simulink model "ALL_JP360_DBW_V6_5_1103"  (R2022a)
settings: Solver=FixedStepAuto  StartTime=0.0  StopTime=inf  FixedStep=0.01  RelTol=1e-3  EnableMultiTasking=on
model workspace (MAT data in the model file):
  g = 9.8
undefined symbols (not defined in the file or in its folder): canChannel, delta_v_p, IPM_Line_C0, IPM_Line_C1, IPM_Line_C2, IPM_Line_C3, M, M_p, MRR_ObjDistX, MRR_ObjDistY, MRR_ObjFusionCamID, MRR_ObjFusionSig, MRR_ObjID, MRR_ObjRelVelX, MRR_ObjRelVelY, MRR_ObjType, MRR_ObjUpdFlg, none, obj_vaild, untracktime, V, videoinput
libraries: canfdmsglib x230, canfdlib x76, slpidlib x24, simulink x18, dspstat3 x14, ctrlSharedLib x1, simulink_extras x1, imaqlib x1, realtime_pacer_lib x1, dspvision x1, visionsinks x1
(part 25 of 55)

== system ALL_JP360_DBW_V6_5_1103/MsgFromCAN/SRR_ADCU_MsgFromCAN/SRR_ADCU_FRR_OBJPos1_0x1A3 ==
  SRR_ADCU_FRR_OBJPos1_0x1A3FromInData : Inport  OutDataTypeStr=Bus:CAN_FD_MESSAGE_BUS
  Bus Creator : BusCreator  Inputs=42  OutDataTypeStr=Bus:SRR_ADCU_FRR_OBJPos1_0x1A3  NonVirtualBus=on
  CAN FD Unpack : canfdmsglib/CAN FD Unpack  CANdbFile=V363 SRR Private CAN-V1.3.dbc  MsgList=(none)  MsgName=FRR_OBJPos1_0x1A3  ProtocolMode=CAN FD  MsgIDType=Standard (11-bit identifier)  MsgIdentifier=419  MsgLength=48  SignalInfo={'FRR_CRCCheck_0x1A3','376','16','BE','unsigned','Standard','0','1','0','0','65535';'FRR_OBJ1_Dx','79','13','BE','unsigned','Standard','0','0.0625','-256','-256','255.938';'FRR_OBJ1_Dy','60','11','BE','unsigned','Standard','0','0.125','-128','-128','127.875';'FRR_OBJ1_ExistProb','112','6','BE','unsigned','Standard','0','2','0','0','100';'FRR_OBJ1_HeadingAngle','55','10','BE','unsigned','Standard','0','0.01','-3.14','-3.14','3.14';'FRR_OBJ1_Height','26','9','BE','unsigned','Standard','0','0.01','0','0','5.11';'FRR_OBJ1_Length','33','9','BE','unsigned','Standard','0','0.05','0','0','25.5';'FRR_OBJ1_Measured','126','2','BE','unsigned','Standard','0','1','0','0','3';'FRR_OBJ1_Motion_Status','162','3','BE','unsigned','Standard','0','1','0','0','7';'FRR_OBJ1_ObstacleProb','120','6','BE','unsigned','Standard','0','2','0','0','100';'FRR_OBJ1_RefPointDx','144','13','BE','unsigned','Standard','0','0.0625','-256','-256','255.938';'FRR_OBJ1_RefPointDy','141','11','BE','unsigned','Standard','0','0.125','-128','-128','127.875';'FRR_OBJ1_RefPointLoc','157','3','BE','unsigned','Standard','0','1','0','0','7';'FRR_OBJ1_RelAx','118','9','BE','unsigned','Standard','0','0.0625','-16','-16','15.9375';'FRR_OBJ1_RelAy','111','10','BE','unsigned','Standard','0','0.03125','-16','-16','15.9688';'FRR_OBJ1_RelVx','89','12','BE','unsigned','Standard','0','0.0625','-128','-128','127.938';'FRR_OBJ1_RelVy','85','10','BE','unsigned','Standard','0','0.125','-64','-64','63.875';'FRR_OBJ1_Track_Age','165','8','BE','unsigned','Standard','0','1','0','0','255';'FRR_OBJ1_Track_ID','1','7','BE','unsigned','Standard','0','1','0','0','127';'FRR_OBJ1_Type','14','3','BE','unsigned','Standard','0','1','0','0','7';'FRR_OBJ1_Width','19','11','BE','unsigned','Standard','0','0.01','0','0','12';'FRR_OBJ2_Dx','247','13','BE','unsigned','Standard','0','0.0625','-256','-256','255.938';'FRR_OBJ2_Dy','228','11','BE','unsigned','Standard','0','0.125','-128','-128','127.875';'FRR_OBJ2_ExistProb','280','6','BE','unsigned','Standard','0','2','0','0','100';'FRR_OBJ2_HeadingAngle','223','10','BE','unsigned','Standard','0','0.01','-3.14','-3.14','3.14';'FRR_OBJ2_Height','194','9','BE','unsigned','Standard','0','0.01','0','0','5.11';'FRR_OBJ2_Length','201','9','BE','unsigned','Standard','0','0.05','0','0','25.5';'FRR_OBJ2_Measured','294','2','BE','unsigned','Standard','0','1','0','0','3';'FRR_OBJ2_Motion_Status','330','3','BE','unsigned','Standard','0','1','0','0','7';'FRR_OBJ2_ObstacleProb','288','6','BE','unsigned','Standard','0','2','0','0','100';'FRR_OBJ2_RefPointDx','312','13','BE','unsigned','Standard','0','0.0625','-256','-256','255.938';'FRR_OBJ2_RefPointDy','309','11','BE','unsigned','Standard','0','0.125','-128','-128','127.875';'FRR_OBJ2_RefPointLoc','325','3','BE','unsigned','Standard','0','1','0','0','7';'FRR_OBJ2_RelAx','286','9','BE','unsigned','Standard','0','0.0625','-16','-16','15.9375';'FRR_OBJ2_RelAy','279','10','BE','unsigned','Standard','0','0.03125','-16','-16','15.9688';'FRR_OBJ2_RelVx','257','12','BE','unsigned','Standard','0','0.0625','-128','-128','127.938';'FRR_OBJ2_RelVy','253','10','BE','unsigned','Standard','0','0.125','-64','-64','63.875';'FRR_OBJ2_Track_Age','333','8','BE','unsigned','Standard','0','1','0','0','255';'FRR_OBJ2_Track_ID','169','7','BE','unsigned','Standard','0','1','0','0','127';'FRR_OBJ2_Type','182','3','BE','unsigned','Standard','0','1','0','0','7';'FRR_OBJ2_Width','187','11','BE','unsigned','Standard','0','0.01','0','0','12';'FRR_RollingCounter_0x1A3','360','4','BE','unsigned','Standard','0','1','0','0','15'}  IDPort=off  TimestampPort=off  ErrorPort=off  RemotePort=off  LengthPort=off  StatusPort=off  BRSPort=off  ESIPort=off  DLCPort=off  ApplyMinMax=off
      settings: SourceProductBaseCode=ME,XP,VN  DataFormat=CANdb specified signals
  Data Type Conversion1 : DataTypeConversion  OutDataTypeStr=uint16  SaturateOnIntegerOverflow=off  RndMeth=Floor
  Data Type Conversion{4,8..10,13,19..20,24,28..30,33,39..40,42} (15 alike) : DataTypeConversion  OutDataTypeStr=int8  SaturateOnIntegerOverflow=off  RndMeth=Floor
  Data Type Conversion{2..3,5..7,11..12,14..17,21..23,25..27,31..32,34..37,41} (24 alike) : DataTypeConversion  OutDataTypeStr=single  SaturateOnIntegerOverflow=off  RndMeth=Floor
  Data Type Conversion18 : DataTypeConversion  OutDataTypeStr=uint8  SaturateOnIntegerOverflow=off  RndMeth=Floor
  Data Type Conversion38 : DataTypeConversion  OutDataTypeStr=uint8  SaturateOnIntegerOverflow=off  RndMeth=Floor
  SRR_ADCU_FRR_OBJPos1_0x1A3FromOutData : Outport  OutDataTypeStr=Bus:SRR_ADCU_FRR_OBJPos1_0x1A3
  wires:
  CAN FD Unpack/1 -> Data Type Conversion1/1
  CAN FD Unpack/2 -> Data Type Conversion2/1
  CAN FD Unpack/3 -> Data Type Conversion3/1
  CAN FD Unpack/4 -> Data Type Conversion4/1
  CAN FD Unpack/5 -> Data Type Conversion5/1
  CAN FD Unpack/6 -> Data Type Conversion6/1
  CAN FD Unpack/7 -> Data Type Conversion7/1
  CAN FD Unpack/8 -> Data Type Conversion8/1
  CAN FD Unpack/9 -> Data Type Conversion9/1
  CAN FD Unpack/10 -> Data Type Conversion10/1
  CAN FD Unpack/11 -> Data Type Conversion11/1
  CAN FD Unpack/12 -> Data Type Conversion12/1
  CAN FD Unpack/13 -> Data Type Conversion13/1
  CAN FD Unpack/14 -> Data Type Conversion14/1
  CAN FD Unpack/15 -> Data Type Conversion15/1
  CAN FD Unpack/16 -> Data Type Conversion16/1
  CAN FD Unpack/17 -> Data Type Conversion17/1
  CAN FD Unpack/18 -> Data Type Conversion18/1
  CAN FD Unpack/19 -> Data Type Conversion19/1
  CAN FD Unpack/20 -> Data Type Conversion20/1
  CAN FD Unpack/21 -> Data Type Conversion21/1
  CAN FD Unpack/22 -> Data Type Conversion22/1
  CAN FD Unpack/23 -> Data Type Conversion23/1
  CAN FD Unpack/24 -> Data Type Conversion24/1
  CAN FD Unpack/25 -> Data Type Conversion25/1
  CAN FD Unpack/26 -> Data Type Conversion26/1
  CAN FD Unpack/27 -> Data Type Conversion27/1
  CAN FD Unpack/28 -> Data Type Conversion28/1
  CAN FD Unpack/29 -> Data Type Conversion29/1
  CAN FD Unpack/30 -> Data Type Conversion30/1
  CAN FD Unpack/31 -> Data Type Conversion31/1
  CAN FD Unpack/32 -> Data Type Conversion32/1
  CAN FD Unpack/33 -> Data Type Conversion33/1
  CAN FD Unpack/34 -> Data Type Conversion34/1
  CAN FD Unpack/35 -> Data Type Conversion35/1
  CAN FD Unpack/36 -> Data Type Conversion36/1
  CAN FD Unpack/37 -> Data Type Conversion37/1
  CAN FD Unpack/38 -> Data Type Conversion38/1
  CAN FD Unpack/39 -> Data Type Conversion39/1
  CAN FD Unpack/40 -> Data Type Conversion40/1
  CAN FD Unpack/41 -> Data Type Conversion41/1
  CAN FD Unpack/42 -> Data Type Conversion42/1
  Data Type Conversion1/1 -> Bus Creator/1  "FRR_CRCCheck_0x1A3"
  Data Type Conversion2/1 -> Bus Creator/2  "FRR_OBJ1_Dx"
  Data Type Conversion3/1 -> Bus Creator/3  "FRR_OBJ1_Dy"
  Data Type Conversion4/1 -> Bus Creator/4  "FRR_OBJ1_ExistProb"
  Data Type Conversion5/1 -> Bus Creator/5  "FRR_OBJ1_HeadingAngle"
  Data Type Conversion6/1 -> Bus Creator/6  "FRR_OBJ1_Height"
  Data Type Conversion7/1 -> Bus Creator/7  "FRR_OBJ1_Length"
  Data Type Conversion8/1 -> Bus Creator/8  "FRR_OBJ1_Measured"
  Data Type Conversion9/1 -> Bus Creator/9  "FRR_OBJ1_Motion_Status"
  Data Type Conversion10/1 -> Bus Creator/10  "FRR_OBJ1_ObstacleProb"
  Data Type Conversion11/1 -> Bus Creator/11  "FRR_OBJ1_RefPointDx"
  Data Type Conversion12/1 -> Bus Creator/12  "FRR_OBJ1_RefPointDy"
  Data Type Conversion13/1 -> Bus Creator/13  "FRR_OBJ1_RefPointLoc"
  Data Type Conversion14/1 -> Bus Creator/14  "FRR_OBJ1_RelAx"
  Data Type Conversion15/1 -> Bus Creator/15  "FRR_OBJ1_RelAy"
  Data Type Conversion16/1 -> Bus Creator/16  "FRR_OBJ1_RelVx"
  Data Type Conversion17/1 -> Bus Creator/17  "FRR_OBJ1_RelVy"
  Data Type Conversion18/1 -> Bus Creator/18  "FRR_OBJ1_Track_Age"
  Data Type Conversion19/1 -> Bus Creator/19  "FRR_OBJ1_Track_ID"
  Data Type Conversion20/1 -> Bus Creator/20  "FRR_OBJ1_Type"
  Data Type Conversion21/1 -> Bus Creator/21  "FRR_OBJ1_Width"
  Data Type Conversion22/1 -> Bus Creator/22  "FRR_OBJ2_Dx"
  Data Type Conversion23/1 -> Bus Creator/23  "FRR_OBJ2_Dy"
  Data Type Conversion24/1 -> Bus Creator/24  "FRR_OBJ2_ExistProb"
  Data Type Conversion25/1 -> Bus Creator/25  "FRR_OBJ2_HeadingAngle"
  Data Type Conversion26/1 -> Bus Creator/26  "FRR_OBJ2_Height"
  Data Type Conversion27/1 -> Bus Creator/27  "FRR_OBJ2_Length"
  Data Type Conversion28/1 -> Bus Creator/28  "FRR_OBJ2_Measured"
  Data Type Conversion29/1 -> Bus Creator/29  "FRR_OBJ2_Motion_Status"
  Data Type Conversion30/1 -> Bus Creator/30  "FRR_OBJ2_ObstacleProb"
  Data Type Conversion31/1 -> Bus Creator/31  "FRR_OBJ2_RefPointDx"
  Data Type Conversion32/1 -> Bus Creator/32  "FRR_OBJ2_RefPointDy"
  Data Type Conversion33/1 -> Bus Creator/33  "FRR_OBJ2_RefPointLoc"
  Data Type Conversion34/1 -> Bus Creator/34  "FRR_OBJ2_RelAx"
  Data Type Conversion35/1 -> Bus Creator/35  "FRR_OBJ2_RelAy"
  Data Type Conversion36/1 -> Bus Creator/36  "FRR_OBJ2_RelVx"
  Data Type Conversion37/1 -> Bus Creator/37  "FRR_OBJ2_RelVy"
  Data Type Conversion38/1 -> Bus Creator/38  "FRR_OBJ2_Track_Age"
  Data Type Conversion39/1 -> Bus Creator/39  "FRR_OBJ2_Track_ID"
  Data Type Conversion40/1 -> Bus Creator/40  "FRR_OBJ2_Type"
  Data Type Conversion41/1 -> Bus Creator/41  "FRR_OBJ2_Width"
  Data Type Conversion42/1 -> Bus Creator/42  "FRR_RollingCounter_0x1A3"
  Bus Creator/1 -> SRR_ADCU_FRR_OBJPos1_0x1A3FromOutData/1  "SRR_ADCU_FRR_OBJPos1_0x1A3FromOutData"
  SRR_ADCU_FRR_OBJPos1_0x1A3FromInData/1 -> CAN FD Unpack/1  "SRR_ADCU_FRR_OBJPos1_0x1A3FromInData"

== system ALL_JP360_DBW_V6_5_1103/MsgFromCAN/SRR_ADCU_MsgFromCAN/SRR_ADCU_FRR_OBJPos2_0x1A4 ==
  SRR_ADCU_FRR_OBJPos2_0x1A4FromInData : Inport  OutDataTypeStr=Bus:CAN_FD_MESSAGE_BUS
  Bus Creator : BusCreator  Inputs=42  OutDataTypeStr=Bus:SRR_ADCU_FRR_OBJPos2_0x1A4  NonVirtualBus=on
  CAN FD Unpack : canfdmsglib/CAN FD Unpack  CANdbFile=V363 SRR Private CAN-V1.3.dbc  MsgList=(none)  MsgName=FRR_OBJPos2_0x1A4  ProtocolMode=CAN FD  MsgIDType=Standard (11-bit identifier)  MsgIdentifier=420  MsgLength=48  SignalInfo={'FRR_CRCCheck_0x1A4','376','16','BE','unsigned','Standard','0','1','0','0','65535';'FRR_OBJ3_Dx','79','13','BE','unsigned','Standard','0','0.0625','-256','-256','255.938';'FRR_OBJ3_Dy','60','11','BE','unsigned','Standard','0','0.125','-128','-128','127.875';'FRR_OBJ3_ExistProb','112','6','BE','unsigned','Standard','0','2','0','0','100';'FRR_OBJ3_HeadingAngle','55','10','BE','unsigned','Standard','0','0.01','-3.14','-3.14','3.14';'FRR_OBJ3_Height','26','9','BE','unsigned','Standard','0','0.01','0','0','5.11';'FRR_OBJ3_Length','33','9','BE','unsigned','Standard','0','0.05','0','0','25.5';'FRR_OBJ3_Measured','126','2','BE','unsigned','Standard','0','1','0','0','3';'FRR_OBJ3_Motion_Status','162','3','BE','unsigned','Standard','0','1','0','0','7';'FRR_OBJ3_ObstacleProb','120','6','BE','unsigned','Standard','0','2','0','0','100';'FRR_OBJ3_RefPointDx','144','13','BE','unsigned','Standard','0','0.0625','-256','-256','255.938';'FRR_OBJ3_RefPointDy','141','11','BE','unsigned','Standard','0','0.125','-128','-128','127.875';'FRR_OBJ3_RefPointLoc','157','3','BE','unsigned','Standard','0','1','0','0','7';'FRR_OBJ3_RelAx','118','9','BE','unsigned','Standard','0','0.0625','-16','-16','15.9375';'FRR_OBJ3_RelAy','111','10','BE','unsigned','Standard','0','0.03125','-16','-16','15.9688';'FRR_OBJ3_RelVx','89','12','BE','unsigned','Standard','0','0.0625','-128','-128','127.938';'FRR_OBJ3_RelVy','85','10','BE','unsigned','Standard','0','0.125','-64','-64','63.875';'FRR_OBJ3_Track_Age','165','8','BE','unsigned','Standard','0','1','0','0','255';'FRR_OBJ3_Track_ID','1','7','BE','unsigned','Standard','0','1','0','0','127';'FRR_OBJ3_Type','14','3','BE','unsigned','Standard','0','1','0','0','7';'FRR_OBJ3_Width','19','11','BE','unsigned','Standard','0','0.01','0','0','12';'FRR_OBJ4_Dx','247','13','BE','unsigned','Standard','0','0.0625','-256','-256','255.938';'FRR_OBJ4_Dy','228','11','BE','unsigned','Standard','0','0.125','-128','-128','127.875';'FRR_OBJ4_ExistProb','280','6','BE','unsigned','Standard','0','2','0','0','100';'FRR_OBJ4_HeadingAngle','223','10','BE','unsigned','Standard','0','0.01','-3.14','-3.14','3.14';'FRR_OBJ4_Height','194','9','BE','unsigned','Standard','0','0.01','0','0','5.11';'FRR_OBJ4_Length','201','9','BE','unsigned','Standard','0','0.05','0','0','25.5';'FRR_OBJ4_Measured','294','2','BE','unsigned','Standard','0','1','0','0','3';'FRR_OBJ4_Motion_Status','330','3','BE','unsigned','Standard','0','1','0','0','7';'FRR_OBJ4_ObstacleProb','288','6','BE','unsigned','Standard','0','2','0','0','100';'FRR_OBJ4_RefPointDx','312','13','BE','unsigned','Standard','0','0.0625','-256','-256','255.938';'FRR_OBJ4_RefPointDy','309','11','BE','unsigned','Standard','0','0.125','-128','-128','127.875';'FRR_OBJ4_RefPointLoc','325','3','BE','unsigned','Standard','0','1','0','0','7';'FRR_OBJ4_RelAx','286','9','BE','unsigned','Standard','0','0.0625','-16','-16','15.9375';'FRR_OBJ4_RelAy','279','10','BE','unsigned','Standard','0','0.03125','-16','-16','15.9688';'FRR_OBJ4_RelVx','257','12','BE','unsigned','Standard','0','0.0625','-128','-128','127.938';'FRR_OBJ4_RelVy','253','10','BE','unsigned','Standard','0','0.125','-64','-64','63.875';'FRR_OBJ4_Track_Age','333','8','BE','unsigned','Standard','0','1','0','0','255';'FRR_OBJ4_Track_ID','169','7','BE','unsigned','Standard','0','1','0','0','127';'FRR_OBJ4_Type','182','3','BE','unsigned','Standard','0','1','0','0','7';'FRR_OBJ4_Width','187','11','BE','unsigned','Standard','0','0.01','0','0','12';'FRR_RollingCounter_0x1A4','360','4','BE','unsigned','Standard','0','1','0','0','15'}  IDPort=off  TimestampPort=off  ErrorPort=off  RemotePort=off  LengthPort=off  StatusPort=off  BRSPort=off  ESIPort=off  DLCPort=off  ApplyMinMax=off
      settings: SourceProductBaseCode=ME,XP,VN  DataFormat=CANdb specified signals
  Data Type Conversion1 : DataTypeConversion  OutDataTypeStr=uint16  SaturateOnIntegerOverflow=off  RndMeth=Floor
  Data Type Conversion{4,8..10,13,19..20,24,28..30,33,39..40,42} (15 alike) : DataTypeConversion  OutDataTypeStr=int8  SaturateOnIntegerOverflow=off  RndMeth=Floor
  Data Type Conversion{2..3,5..7,11..12,14..17,21..23,25..27,31..32,34..37,41} (24 alike) : DataTypeConversion  OutDataTypeStr=single  SaturateOnIntegerOverflow=off  RndMeth=Floor
  Data Type Conversion18 : DataTypeConversion  OutDataTypeStr=uint8  SaturateOnIntegerOverflow=off  RndMeth=Floor
  Data Type Conversion38 : DataTypeConversion  OutDataTypeStr=uint8  SaturateOnIntegerOverflow=off  RndMeth=Floor
  SRR_ADCU_FRR_OBJPos2_0x1A4FromOutData : Outport  OutDataTypeStr=Bus:SRR_ADCU_FRR_OBJPos2_0x1A4
  wires:
  CAN FD Unpack/1 -> Data Type Conversion1/1
  CAN FD Unpack/2 -> Data Type Conversion2/1
  CAN FD Unpack/3 -> Data Type Conversion3/1
  CAN FD Unpack/4 -> Data Type Conversion4/1
  CAN FD Unpack/5 -> Data Type Conversion5/1
  CAN FD Unpack/6 -> Data Type Conversion6/1
  CAN FD Unpack/7 -> Data Type Conversion7/1
  CAN FD Unpack/8 -> Data Type Conversion8/1
  CAN FD Unpack/9 -> Data Type Conversion9/1
  CAN FD Unpack/10 -> Data Type Conversion10/1
  CAN FD Unpack/11 -> Data Type Conversion11/1
  CAN FD Unpack/12 -> Data Type Conversion12/1
  CAN FD Unpack/13 -> Data Type Conversion13/1
  CAN FD Unpack/14 -> Data Type Conversion14/1
  CAN FD Unpack/15 -> Data Type Conversion15/1
  CAN FD Unpack/16 -> Data Type Conversion16/1
  CAN FD Unpack/17 -> Data Type Conversion17/1
  CAN FD Unpack/18 -> Data Type Conversion18/1
  CAN FD Unpack/19 -> Data Type Conversion19/1
  CAN FD Unpack/20 -> Data Type Conversion20/1
  CAN FD Unpack/21 -> Data Type Conversion21/1
  CAN FD Unpack/22 -> Data Type Conversion22/1
  CAN FD Unpack/23 -> Data Type Conversion23/1
  CAN FD Unpack/24 -> Data Type Conversion24/1
  CAN FD Unpack/25 -> Data Type Conversion25/1
  CAN FD Unpack/26 -> Data Type Conversion26/1
  CAN FD Unpack/27 -> Data Type Conversion27/1
  CAN FD Unpack/28 -> Data Type Conversion28/1
  CAN FD Unpack/29 -> Data Type Conversion29/1
  CAN FD Unpack/30 -> Data Type Conversion30/1
  CAN FD Unpack/31 -> Data Type Conversion31/1
  CAN FD Unpack/32 -> Data Type Conversion32/1
  CAN FD Unpack/33 -> Data Type Conversion33/1
  CAN FD Unpack/34 -> Data Type Conversion34/1
  CAN FD Unpack/35 -> Data Type Conversion35/1
  CAN FD Unpack/36 -> Data Type Conversion36/1
  CAN FD Unpack/37 -> Data Type Conversion37/1
  CAN FD Unpack/38 -> Data Type Conversion38/1
  CAN FD Unpack/39 -> Data Type Conversion39/1
  CAN FD Unpack/40 -> Data Type Conversion40/1
  CAN FD Unpack/41 -> Data Type Conversion41/1
  CAN FD Unpack/42 -> Data Type Conversion42/1
  Data Type Conversion1/1 -> Bus Creator/1  "FRR_CRCCheck_0x1A4"
  Data Type Conversion2/1 -> Bus Creator/2  "FRR_OBJ3_Dx"
  Data Type Conversion3/1 -> Bus Creator/3  "FRR_OBJ3_Dy"
  Data Type Conversion4/1 -> Bus Creator/4  "FRR_OBJ3_ExistProb"
  Data Type Conversion5/1 -> Bus Creator/5  "FRR_OBJ3_HeadingAngle"
  Data Type Conversion6/1 -> Bus Creator/6  "FRR_OBJ3_Height"
  Data Type Conversion7/1 -> Bus Creator/7  "FRR_OBJ3_Length"
  Data Type Conversion8/1 -> Bus Creator/8  "FRR_OBJ3_Measured"
  Data Type Conversion9/1 -> Bus Creator/9  "FRR_OBJ3_Motion_Status"
  Data Type Conversion10/1 -> Bus Creator/10  "FRR_OBJ3_ObstacleProb"
  Data Type Conversion11/1 -> Bus Creator/11  "FRR_OBJ3_RefPointDx"
  Data Type Conversion12/1 -> Bus Creator/12  "FRR_OBJ3_RefPointDy"
  Data Type Conversion13/1 -> Bus Creator/13  "FRR_OBJ3_RefPointLoc"
  Data Type Conversion14/1 -> Bus Creator/14  "FRR_OBJ3_RelAx"
  Data Type Conversion15/1 -> Bus Creator/15  "FRR_OBJ3_RelAy"
  Data Type Conversion16/1 -> Bus Creator/16  "FRR_OBJ3_RelVx"
  Data Type Conversion17/1 -> Bus Creator/17  "FRR_OBJ3_RelVy"
  Data Type Conversion18/1 -> Bus Creator/18  "FRR_OBJ3_Track_Age"
  Data Type Conversion19/1 -> Bus Creator/19  "FRR_OBJ3_Track_ID"
  Data Type Conversion20/1 -> Bus Creator/20  "FRR_OBJ3_Type"
  Data Type Conversion21/1 -> Bus Creator/21  "FRR_OBJ3_Width"
  Data Type Conversion22/1 -> Bus Creator/22  "FRR_OBJ4_Dx"
  Data Type Conversion23/1 -> Bus Creator/23  "FRR_OBJ4_Dy"
  Data Type Conversion24/1 -> Bus Creator/24  "FRR_OBJ4_ExistProb"
  Data Type Conversion25/1 -> Bus Creator/25  "FRR_OBJ4_HeadingAngle"
  Data Type Conversion26/1 -> Bus Creator/26  "FRR_OBJ4_Height"
  Data Type Conversion27/1 -> Bus Creator/27  "FRR_OBJ4_Length"
  Data Type Conversion28/1 -> Bus Creator/28  "FRR_OBJ4_Measured"
  Data Type Conversion29/1 -> Bus Creator/29  "FRR_OBJ4_Motion_Status"
  Data Type Conversion30/1 -> Bus Creator/30  "FRR_OBJ4_ObstacleProb"
  Data Type Conversion31/1 -> Bus Creator/31  "FRR_OBJ4_RefPointDx"
  Data Type Conversion32/1 -> Bus Creator/32  "FRR_OBJ4_RefPointDy"
  Data Type Conversion33/1 -> Bus Creator/33  "FRR_OBJ4_RefPointLoc"
  Data Type Conversion34/1 -> Bus Creator/34  "FRR_OBJ4_RelAx"
  Data Type Conversion35/1 -> Bus Creator/35  "FRR_OBJ4_RelAy"
  Data Type Conversion36/1 -> Bus Creator/36  "FRR_OBJ4_RelVx"
  Data Type Conversion37/1 -> Bus Creator/37  "FRR_OBJ4_RelVy"
  Data Type Conversion38/1 -> Bus Creator/38  "FRR_OBJ4_Track_Age"
  Data Type Conversion39/1 -> Bus Creator/39  "FRR_OBJ4_Track_ID"
  Data Type Conversion40/1 -> Bus Creator/40  "FRR_OBJ4_Type"
  Data Type Conversion41/1 -> Bus Creator/41  "FRR_OBJ4_Width"
  Data Type Conversion42/1 -> Bus Creator/42  "FRR_RollingCounter_0x1A4"
  Bus Creator/1 -> SRR_ADCU_FRR_OBJPos2_0x1A4FromOutData/1  "SRR_ADCU_FRR_OBJPos2_0x1A4FromOutData"
  SRR_ADCU_FRR_OBJPos2_0x1A4FromInData/1 -> CAN FD Unpack/1  "SRR_ADCU_FRR_OBJPos2_0x1A4FromInData"

== system ALL_JP360_DBW_V6_5_1103/MsgFromCAN/SRR_ADCU_MsgFromCAN/SRR_ADCU_FRR_OBJPos3_0x1A5 ==
  SRR_ADCU_FRR_OBJPos3_0x1A5FromInData : Inport  OutDataTypeStr=Bus:CAN_FD_MESSAGE_BUS
  Bus Creator : BusCreator  Inputs=42  OutDataTypeStr=Bus:SRR_ADCU_FRR_OBJPos3_0x1A5  NonVirtualBus=on
  CAN FD Unpack : canfdmsglib/CAN FD Unpack  CANdbFile=V363 SRR Private CAN-V1.3.dbc  MsgList=(none)  MsgName=FRR_OBJPos3_0x1A5  ProtocolMode=CAN FD  MsgIDType=Standard (11-bit identifier)  MsgIdentifier=421  MsgLength=48  SignalInfo={'FRR_CRCCheck_0x1A5','376','16','BE','unsigned','Standard','0','1','0','0','65535';'FRR_OBJ5_Dx','79','13','BE','unsigned','Standard','0','0.0625','-256','-256','255.938';'FRR_OBJ5_Dy','60','11','BE','unsigned','Standard','0','0.125','-128','-128','127.875';'FRR_OBJ5_ExistProb','112','6','BE','unsigned','Standard','0','2','0','0','100';'FRR_OBJ5_HeadingAngle','55','10','BE','unsigned','Standard','0','0.01','-3.14','-3.14','3.14';'FRR_OBJ5_Height','26','9','BE','unsigned','Standard','0','0.01','0','0','5.11';'FRR_OBJ5_Length','33','9','BE','unsigned','Standard','0','0.05','0','0','25.5';'FRR_OBJ5_Measured','126','2','BE','unsigned','Standard','0','1','0','0','3';'FRR_OBJ5_Motion_Status','162','3','BE','unsigned','Standard','0','1','0','0','7';'FRR_OBJ5_ObstacleProb','120','6','BE','unsigned','Standard','0','2','0','0','100';'FRR_OBJ5_RefPointDx','144','13','BE','unsigned','Standard','0','0.0625','-256','-256','255.938';'FRR_OBJ5_RefPointDy','141','11','BE','unsigned','Standard','0','0.125','-128','-128','127.875';'FRR_OBJ5_RefPointLoc','157','3','BE','unsigned','Standard','0','1','0','0','7';'FRR_OBJ5_RelAx','118','9','BE','unsigned','Standard','0','0.0625','-16','-16','15.9375';'FRR_OBJ5_RelAy','111','10','BE','unsigned','Standard','0','0.03125','-16','-16','15.9688';'FRR_OBJ5_RelVx','89','12','BE','unsigned','Standard','0','0.0625','-128','-128','127.938';'FRR_OBJ5_RelVy','85','10','BE','unsigned','Standard','0','0.125','-64','-64','63.875';'FRR_OBJ5_Track_Age','165','8','BE','unsigned','Standard','0','1','0','0','255';'FRR_OBJ5_Track_ID','1','7','BE','unsigned','Standard','0','1','0','0','127';'FRR_OBJ5_Type','14','3','BE','unsigned','Standard','0','1','0','0','7';'FRR_OBJ5_Width','19','11','BE','unsigned','Standard','0','0.01','0','0','12';'FRR_OBJ6_Dx','247','13','BE','unsigned','Standard','0','0.0625','-256','-256','255.938';'FRR_OBJ6_Dy','228','11','BE','unsigned','Standard','0','0.125','-128','-128','127.875';'FRR_OBJ6_ExistProb','280','6','BE','unsigned','Standard','0','2','0','0','100';'FRR_OBJ6_HeadingAngle','223','10','BE','unsigned','Standard','0','0.01','-3.14','-3.14','3.14';'FRR_OBJ6_Height','194','9','BE','unsigned','Standard','0','0.01','0','0','5.11';'FRR_OBJ6_Length','201','9','BE','unsigned','Standard','0','0.05','0','0','25.5';'FRR_OBJ6_Measured','294','2','BE','unsigned','Standard','0','1','0','0','3';'FRR_OBJ6_Motion_Status','330','3','BE','unsigned','Standard','0','1','0','0','7';'FRR_OBJ6_ObstacleProb','288','6','BE','unsigned','Standard','0','2','0','0','100';'FRR_OBJ6_RefPointDx','312','13','BE','unsigned','Standard','0','0.0625','-256','-256','255.938';'FRR_OBJ6_RefPointDy','309','11','BE','unsigned','Standard','0','0.125','-128','-128','127.875';'FRR_OBJ6_RefPointLoc','325','3','BE','unsigned','Standard','0','1','0','0','7';'FRR_OBJ6_RelAx','286','9','BE','unsigned','Standard','0','0.0625','-16','-16','15.9375';'FRR_OBJ6_RelAy','279','10','BE','unsigned','Standard','0','0.03125','-16','-16','15.9688';'FRR_OBJ6_RelVx','257','12','BE','unsigned','Standard','0','0.0625','-128','-128','127.938';'FRR_OBJ6_RelVy','253','10','BE','unsigned','Standard','0','0.125','-64','-64','63.875';'FRR_OBJ6_Track_Age','333','8','BE','unsigned','Standard','0','1','0','0','255';'FRR_OBJ6_Track_ID','169','7','BE','unsigned','Standard','0','1','0','0','127';'FRR_OBJ6_Type','182','3','BE','unsigned','Standard','0','1','0','0','7';'FRR_OBJ6_Width','187','11','BE','unsigned','Standard','0','0.01','0','0','12';'FRR_RollingCounter_0x1A5','360','4','BE','unsigned','Standard','0','1','0','0','15'}  IDPort=off  TimestampPort=off  ErrorPort=off  RemotePort=off  LengthPort=off  StatusPort=off  BRSPort=off  ESIPort=off  DLCPort=off  ApplyMinMax=off
      settings: SourceProductBaseCode=ME,XP,VN  DataFormat=CANdb specified signals
  Data Type Conversion1 : DataTypeConversion  OutDataTypeStr=uint16  SaturateOnIntegerOverflow=off  RndMeth=Floor
  Data Type Conversion{4,8..10,13,19..20,24,28..30,33,39..40,42} (15 alike) : DataTypeConversion  OutDataTypeStr=int8  SaturateOnIntegerOverflow=off  RndMeth=Floor
  Data Type Conversion{2..3,5..7,11..12,14..17,21..23,25..27,31..32,34..37,41} (24 alike) : DataTypeConversion  OutDataTypeStr=single  SaturateOnIntegerOverflow=off  RndMeth=Floor
  Data Type Conversion18 : DataTypeConversion  OutDataTypeStr=uint8  SaturateOnIntegerOverflow=off  RndMeth=Floor
  Data Type Conversion38 : DataTypeConversion  OutDataTypeStr=uint8  SaturateOnIntegerOverflow=off  RndMeth=Floor
  SRR_ADCU_FRR_OBJPos3_0x1A5FromOutData : Outport  OutDataTypeStr=Bus:SRR_ADCU_FRR_OBJPos3_0x1A5
  wires:
  CAN FD Unpack/1 -> Data Type Conversion1/1
  CAN FD Unpack/2 -> Data Type Conversion2/1
  CAN FD Unpack/3 -> Data Type Conversion3/1
  CAN FD Unpack/4 -> Data Type Conversion4/1
  CAN FD Unpack/5 -> Data Type Conversion5/1
  CAN FD Unpack/6 -> Data Type Conversion6/1
  CAN FD Unpack/7 -> Data Type Conversion7/1
  CAN FD Unpack/8 -> Data Type Conversion8/1
  CAN FD Unpack/9 -> Data Type Conversion9/1
  CAN FD Unpack/10 -> Data Type Conversion10/1
  CAN FD Unpack/11 -> Data Type Conversion11/1
  CAN FD Unpack/12 -> Data Type Conversion12/1
  CAN FD Unpack/13 -> Data Type Conversion13/1
  CAN FD Unpack/14 -> Data Type Conversion14/1
  CAN FD Unpack/15 -> Data Type Conversion15/1
  CAN FD Unpack/16 -> Data Type Conversion16/1
  CAN FD Unpack/17 -> Data Type Conversion17/1
  CAN FD Unpack/18 -> Data Type Conversion18/1
  CAN FD Unpack/19 -> Data Type Conversion19/1
  CAN FD Unpack/20 -> Data Type Conversion20/1
  CAN FD Unpack/21 -> Data Type Conversion21/1
  CAN FD Unpack/22 -> Data Type Conversion22/1
  CAN FD Unpack/23 -> Data Type Conversion23/1
  CAN FD Unpack/24 -> Data Type Conversion24/1
  CAN FD Unpack/25 -> Data Type Conversion25/1
  CAN FD Unpack/26 -> Data Type Conversion26/1
  CAN FD Unpack/27 -> Data Type Conversion27/1
  CAN FD Unpack/28 -> Data Type Conversion28/1
  CAN FD Unpack/29 -> Data Type Conversion29/1
  CAN FD Unpack/30 -> Data Type Conversion30/1
  CAN FD Unpack/31 -> Data Type Conversion31/1
  CAN FD Unpack/32 -> Data Type Conversion32/1
  CAN FD Unpack/33 -> Data Type Conversion33/1
  CAN FD Unpack/34 -> Data Type Conversion34/1
  CAN FD Unpack/35 -> Data Type Conversion35/1
  CAN FD Unpack/36 -> Data Type Conversion36/1
  CAN FD Unpack/37 -> Data Type Conversion37/1
  CAN FD Unpack/38 -> Data Type Conversion38/1
  CAN FD Unpack/39 -> Data Type Conversion39/1
  CAN FD Unpack/40 -> Data Type Conversion40/1
  CAN FD Unpack/41 -> Data Type Conversion41/1
  CAN FD Unpack/42 -> Data Type Conversion42/1
  Data Type Conversion1/1 -> Bus Creator/1  "FRR_CRCCheck_0x1A5"
  Data Type Conversion2/1 -> Bus Creator/2  "FRR_OBJ5_Dx"
  Data Type Conversion3/1 -> Bus Creator/3  "FRR_OBJ5_Dy"
  Data Type Conversion4/1 -> Bus Creator/4  "FRR_OBJ5_ExistProb"
  Data Type Conversion5/1 -> Bus Creator/5  "FRR_OBJ5_HeadingAngle"
  Data Type Conversion6/1 -> Bus Creator/6  "FRR_OBJ5_Height"
  Data Type Conversion7/1 -> Bus Creator/7  "FRR_OBJ5_Length"
  Data Type Conversion8/1 -> Bus Creator/8  "FRR_OBJ5_Measured"
  Data Type Conversion9/1 -> Bus Creator/9  "FRR_OBJ5_Motion_Status"
  Data Type Conversion10/1 -> Bus Creator/10  "FRR_OBJ5_ObstacleProb"
  Data Type Conversion11/1 -> Bus Creator/11  "FRR_OBJ5_RefPointDx"
  Data Type Conversion12/1 -> Bus Creator/12  "FRR_OBJ5_RefPointDy"
  Data Type Conversion13/1 -> Bus Creator/13  "FRR_OBJ5_RefPointLoc"
  Data Type Conversion14/1 -> Bus Creator/14  "FRR_OBJ5_RelAx"
  Data Type Conversion15/1 -> Bus Creator/15  "FRR_OBJ5_RelAy"
  Data Type Conversion16/1 -> Bus Creator/16  "FRR_OBJ5_RelVx"
  Data Type Conversion17/1 -> Bus Creator/17  "FRR_OBJ5_RelVy"
  Data Type Conversion18/1 -> Bus Creator/18  "FRR_OBJ5_Track_Age"
  Data Type Conversion19/1 -> Bus Creator/19  "FRR_OBJ5_Track_ID"
  Data Type Conversion20/1 -> Bus Creator/20  "FRR_OBJ5_Type"
  Data Type Conversion21/1 -> Bus Creator/21  "FRR_OBJ5_Width"
  Data Type Conversion22/1 -> Bus Creator/22  "FRR_OBJ6_Dx"
  Data Type Conversion23/1 -> Bus Creator/23  "FRR_OBJ6_Dy"
  Data Type Conversion24/1 -> Bus Creator/24  "FRR_OBJ6_ExistProb"
  Data Type Conversion25/1 -> Bus Creator/25  "FRR_OBJ6_HeadingAngle"
  Data Type Conversion26/1 -> Bus Creator/26  "FRR_OBJ6_Height"
  Data Type Conversion27/1 -> Bus Creator/27  "FRR_OBJ6_Length"
  Data Type Conversion28/1 -> Bus Creator/28  "FRR_OBJ6_Measured"
  Data Type Conversion29/1 -> Bus Creator/29  "FRR_OBJ6_Motion_Status"
  Data Type Conversion30/1 -> Bus Creator/30  "FRR_OBJ6_ObstacleProb"
  Data Type Conversion31/1 -> Bus Creator/31  "FRR_OBJ6_RefPointDx"
  Data Type Conversion32/1 -> Bus Creator/32  "FRR_OBJ6_RefPointDy"
  Data Type Conversion33/1 -> Bus Creator/33  "FRR_OBJ6_RefPointLoc"
  Data Type Conversion34/1 -> Bus Creator/34  "FRR_OBJ6_RelAx"
  Data Type Conversion35/1 -> Bus Creator/35  "FRR_OBJ6_RelAy"
  Data Type Conversion36/1 -> Bus Creator/36  "FRR_OBJ6_RelVx"
  Data Type Conversion37/1 -> Bus Creator/37  "FRR_OBJ6_RelVy"
  Data Type Conversion38/1 -> Bus Creator/38  "FRR_OBJ6_Track_Age"
  Data Type Conversion39/1 -> Bus Creator/39  "FRR_OBJ6_Track_ID"
  Data Type Conversion40/1 -> Bus Creator/40  "FRR_OBJ6_Type"
  Data Type Conversion41/1 -> Bus Creator/41  "FRR_OBJ6_Width"
  Data Type Conversion42/1 -> Bus Creator/42  "FRR_RollingCounter_0x1A5"
  Bus Creator/1 -> SRR_ADCU_FRR_OBJPos3_0x1A5FromOutData/1  "SRR_ADCU_FRR_OBJPos3_0x1A5FromOutData"
  SRR_ADCU_FRR_OBJPos3_0x1A5FromInData/1 -> CAN FD Unpack/1  "SRR_ADCU_FRR_OBJPos3_0x1A5FromInData"

== system ALL_JP360_DBW_V6_5_1103/MsgFromCAN/SRR_ADCU_MsgFromCAN/SRR_ADCU_FRR_OBJPos4_0x1A6 ==
  SRR_ADCU_FRR_OBJPos4_0x1A6FromInData : Inport  OutDataTypeStr=Bus:CAN_FD_MESSAGE_BUS
  Bus Creator : BusCreator  Inputs=42  OutDataTypeStr=Bus:SRR_ADCU_FRR_OBJPos4_0x1A6  NonVirtualBus=on
  CAN FD Unpack : canfdmsglib/CAN FD Unpack  CANdbFile=V363 SRR Private CAN-V1.3.dbc  MsgList=(none)  MsgName=FRR_OBJPos4_0x1A6  ProtocolMode=CAN FD  MsgIDType=Standard (11-bit identifier)  MsgIdentifier=422  MsgLength=48  SignalInfo={'FRR_CRCCheck_0x1A6','376','16','BE','unsigned','Standard','0','1','0','0','65535';'FRR_OBJ7_Dx','79','13','BE','unsigned','Standard','0','0.0625','-256','-256','255.938';'FRR_OBJ7_Dy','60','11','BE','unsigned','Standard','0','0.125','-128','-128','127.875';'FRR_OBJ7_ExistProb','112','6','BE','unsigned','Standard','0','2','0','0','100';'FRR_OBJ7_HeadingAngle','55','10','BE','unsigned','Standard','0','0.01','-3.14','-3.14','3.14';'FRR_OBJ7_Height','26','9','BE','unsigned','Standard','0','0.01','0','0','5.11';'FRR_OBJ7_Length','33','9','BE','unsigned','Standard','0','0.05','0','0','25.5';'FRR_OBJ7_Measured','126','2','BE','unsigned','Standard','0','1','0','0','3';'FRR_OBJ7_Motion_Status','162','3','BE','unsigned','Standard','0','1','0','0','7';'FRR_OBJ7_ObstacleProb','120','6','BE','unsigned','Standard','0','2','0','0','100';'FRR_OBJ7_RefPointDx','144','13','BE','unsigned','Standard','0','0.0625','-256','-256','255.938';'FRR_OBJ7_RefPointDy','141','11','BE','unsigned','Standard','0','0.125','-128','-128','127.875';'FRR_OBJ7_RefPointLoc','157','3','BE','unsigned','Standard','0','1','0','0','7';'FRR_OBJ7_RelAx','118','9','BE','unsigned','Standard','0','0.0625','-16','-16','15.9375';'FRR_OBJ7_RelAy','111','10','BE','unsigned','Standard','0','0.03125','-16','-16','15.9688';'FRR_OBJ7_RelVx','89','12','BE','unsigned','Standard','0','0.0625','-128','-128','127.938';'FRR_OBJ7_RelVy','85','10','BE','unsigned','Standard','0','0.125','-64','-64','63.875';'FRR_OBJ7_Track_Age','165','8','BE','unsigned','Standard','0','1','0','0','255';'FRR_OBJ7_Track_ID','1','7','BE','unsigned','Standard','0','1','0','0','127';'FRR_OBJ7_Type','14','3','BE','unsigned','Standard','0','1','0','0','7';'FRR_OBJ7_Width','19','11','BE','unsigned','Standard','0','0.01','0','0','12';'FRR_OBJ8_Dx','247','13','BE','unsigned','Standard','0','0.0625','-256','-256','255.938';'FRR_OBJ8_Dy','228','11','BE','unsigned','Standard','0','0.125','-128','-128','127.875';'FRR_OBJ8_ExistProb','280','6','BE','unsigned','Standard','0','2','0','0','100';'FRR_OBJ8_HeadingAngle','223','10','BE','unsigned','Standard','0','0.01','-3.14','-3.14','3.14';'FRR_OBJ8_Height','194','9','BE','unsigned','Standard','0','0.01','0','0','5.11';'FRR_OBJ8_Length','201','9','BE','unsigned','Standard','0','0.05','0','0','25.5';'FRR_OBJ8_Measured','294','2','BE','unsigned','Standard','0','1','0','0','3';'FRR_OBJ8_Motion_Status','330','3','BE','unsigned','Standard','0','1','0','0','7';'FRR_OBJ8_ObstacleProb','288','6','BE','unsigned','Standard','0','2','0','0','100';'FRR_OBJ8_RefPointDx','312','13','BE','unsigned','Standard','0','0.0625','-256','-256','255.938';'FRR_OBJ8_RefPointDy','309','11','BE','unsigned','Standard','0','0.125','-128','-128','127.875';'FRR_OBJ8_RefPointLoc','325','3','BE','unsigned','Standard','0','1','0','0','7';'FRR_OBJ8_RelAx','286','9','BE','unsigned','Standard','0','0.0625','-16','-16','15.9375';'FRR_OBJ8_RelAy','279','10','BE','unsigned','Standard','0','0.03125','-16','-16','15.9688';'FRR_OBJ8_RelVx','257','12','BE','unsigned','Standard','0','0.0625','-128','-128','127.938';'FRR_OBJ8_RelVy','253','10','BE','unsigned','Standard','0','0.125','-64','-64','63.875';'FRR_OBJ8_Track_Age','333','8','BE','unsigned','Standard','0','1','0','0','255';'FRR_OBJ8_Track_ID','169','7','BE','unsigned','Standard','0','1','0','0','127';'FRR_OBJ8_Type','182','3','BE','unsigned','Standard','0','1','0','0','7';'FRR_OBJ8_Width','187','11','BE','unsigned','Standard','0','0.01','0','0','12';'FRR_RollingCounter_0x1A6','360','4','BE','unsigned','Standard','0','1','0','0','15'}  IDPort=off  TimestampPort=off  ErrorPort=off  RemotePort=off  LengthPort=off  StatusPort=off  BRSPort=off  ESIPort=off  DLCPort=off  ApplyMinMax=off
      settings: SourceProductBaseCode=ME,XP,VN  DataFormat=CANdb specified signals
  Data Type Conversion1 : DataTypeConversion  OutDataTypeStr=uint16  SaturateOnIntegerOverflow=off  RndMeth=Floor
  Data Type Conversion{4,8..10,13,19..20,24,28..30,33,39..40,42} (15 alike) : DataTypeConversion  OutDataTypeStr=int8  SaturateOnIntegerOverflow=off  RndMeth=Floor
  Data Type Conversion{2..3,5..7,11..12,14..17,21..23,25..27,31..32,34..37,41} (24 alike) : DataTypeConversion  OutDataTypeStr=single  SaturateOnIntegerOverflow=off  RndMeth=Floor
  Data Type Conversion18 : DataTypeConversion  OutDataTypeStr=uint8  SaturateOnIntegerOverflow=off  RndMeth=Floor
  Data Type Conversion38 : DataTypeConversion  OutDataTypeStr=uint8  SaturateOnIntegerOverflow=off  RndMeth=Floor
  SRR_ADCU_FRR_OBJPos4_0x1A6FromOutData : Outport  OutDataTypeStr=Bus:SRR_ADCU_FRR_OBJPos4_0x1A6
  wires:
  CAN FD Unpack/1 -> Data Type Conversion1/1
  CAN FD Unpack/2 -> Data Type Conversion2/1
  CAN FD Unpack/3 -> Data Type Conversion3/1
  CAN FD Unpack/4 -> Data Type Conversion4/1
  CAN FD Unpack/5 -> Data Type Conversion5/1
  CAN FD Unpack/6 -> Data Type Conversion6/1
  CAN FD Unpack/7 -> Data Type Conversion7/1
  CAN FD Unpack/8 -> Data Type Conversion8/1
  CAN FD Unpack/9 -> Data Type Conversion9/1
  CAN FD Unpack/10 -> Data Type Conversion10/1
  CAN FD Unpack/11 -> Data Type Conversion11/1
  CAN FD Unpack/12 -> Data Type Conversion12/1
  CAN FD Unpack/13 -> Data Type Conversion13/1
  CAN FD Unpack/14 -> Data Type Conversion14/1
  CAN FD Unpack/15 -> Data Type Conversion15/1
  CAN FD Unpack/16 -> Data Type Conversion16/1
  CAN FD Unpack/17 -> Data Type Conversion17/1
  CAN FD Unpack/18 -> Data Type Conversion18/1
  CAN FD Unpack/19 -> Data Type Conversion19/1
  CAN FD Unpack/20 -> Data Type Conversion20/1
  CAN FD Unpack/21 -> Data Type Conversion21/1
  CAN FD Unpack/22 -> Data Type Conversion22/1
  CAN FD Unpack/23 -> Data Type Conversion23/1
  CAN FD Unpack/24 -> Data Type Conversion24/1
  CAN FD Unpack/25 -> Data Type Conversion25/1
  CAN FD Unpack/26 -> Data Type Conversion26/1
  CAN FD Unpack/27 -> Data Type Conversion27/1
  CAN FD Unpack/28 -> Data Type Conversion28/1
  CAN FD Unpack/29 -> Data Type Conversion29/1
  CAN FD Unpack/30 -> Data Type Conversion30/1
  CAN FD Unpack/31 -> Data Type Conversion31/1
  CAN FD Unpack/32 -> Data Type Conversion32/1
  CAN FD Unpack/33 -> Data Type Conversion33/1
  CAN FD Unpack/34 -> Data Type Conversion34/1
  CAN FD Unpack/35 -> Data Type Conversion35/1
  CAN FD Unpack/36 -> Data Type Conversion36/1
  CAN FD Unpack/37 -> Data Type Conversion37/1
  CAN FD Unpack/38 -> Data Type Conversion38/1
  CAN FD Unpack/39 -> Data Type Conversion39/1
  CAN FD Unpack/40 -> Data Type Conversion40/1
  CAN FD Unpack/41 -> Data Type Conversion41/1
  CAN FD Unpack/42 -> Data Type Conversion42/1
  Data Type Conversion1/1 -> Bus Creator/1  "FRR_CRCCheck_0x1A6"
  Data Type Conversion2/1 -> Bus Creator/2  "FRR_OBJ7_Dx"
  Data Type Conversion3/1 -> Bus Creator/3  "FRR_OBJ7_Dy"
  Data Type Conversion4/1 -> Bus Creator/4  "FRR_OBJ7_ExistProb"
  Data Type Conversion5/1 -> Bus Creator/5  "FRR_OBJ7_HeadingAngle"
  Data Type Conversion6/1 -> Bus Creator/6  "FRR_OBJ7_Height"
  Data Type Conversion7/1 -> Bus Creator/7  "FRR_OBJ7_Length"
  Data Type Conversion8/1 -> Bus Creator/8  "FRR_OBJ7_Measured"
  Data Type Conversion9/1 -> Bus Creator/9  "FRR_OBJ7_Motion_Status"
  Data Type Conversion10/1 -> Bus Creator/10  "FRR_OBJ7_ObstacleProb"
  Data Type Conversion11/1 -> Bus Creator/11  "FRR_OBJ7_RefPointDx"
  Data Type Conversion12/1 -> Bus Creator/12  "FRR_OBJ7_RefPointDy"
  Data Type Conversion13/1 -> Bus Creator/13  "FRR_OBJ7_RefPointLoc"
  Data Type Conversion14/1 -> Bus Creator/14  "FRR_OBJ7_RelAx"
  Data Type Conversion15/1 -> Bus Creator/15  "FRR_OBJ7_RelAy"
  Data Type Conversion16/1 -> Bus Creator/16  "FRR_OBJ7_RelVx"
  Data Type Conversion17/1 -> Bus Creator/17  "FRR_OBJ7_RelVy"
  Data Type Conversion18/1 -> Bus Creator/18  "FRR_OBJ7_Track_Age"
  Data Type Conversion19/1 -> Bus Creator/19  "FRR_OBJ7_Track_ID"
  Data Type Conversion20/1 -> Bus Creator/20  "FRR_OBJ7_Type"
  Data Type Conversion21/1 -> Bus Creator/21  "FRR_OBJ7_Width"
  Data Type Conversion22/1 -> Bus Creator/22  "FRR_OBJ8_Dx"
  Data Type Conversion23/1 -> Bus Creator/23  "FRR_OBJ8_Dy"
  Data Type Conversion24/1 -> Bus Creator/24  "FRR_OBJ8_ExistProb"
  Data Type Conversion25/1 -> Bus Creator/25  "FRR_OBJ8_HeadingAngle"
  Data Type Conversion26/1 -> Bus Creator/26  "FRR_OBJ8_Height"
  Data Type Conversion27/1 -> Bus Creator/27  "FRR_OBJ8_Length"
  Data Type Conversion28/1 -> Bus Creator/28  "FRR_OBJ8_Measured"
  Data Type Conversion29/1 -> Bus Creator/29  "FRR_OBJ8_Motion_Status"
  Data Type Conversion30/1 -> Bus Creator/30  "FRR_OBJ8_ObstacleProb"
  Data Type Conversion31/1 -> Bus Creator/31  "FRR_OBJ8_RefPointDx"
  Data Type Conversion32/1 -> Bus Creator/32  "FRR_OBJ8_RefPointDy"
  Data Type Conversion33/1 -> Bus Creator/33  "FRR_OBJ8_RefPointLoc"
  Data Type Conversion34/1 -> Bus Creator/34  "FRR_OBJ8_RelAx"
  Data Type Conversion35/1 -> Bus Creator/35  "FRR_OBJ8_RelAy"
  Data Type Conversion36/1 -> Bus Creator/36  "FRR_OBJ8_RelVx"
  Data Type Conversion37/1 -> Bus Creator/37  "FRR_OBJ8_RelVy"
  Data Type Conversion38/1 -> Bus Creator/38  "FRR_OBJ8_Track_Age"
  Data Type Conversion39/1 -> Bus Creator/39  "FRR_OBJ8_Track_ID"
  Data Type Conversion40/1 -> Bus Creator/40  "FRR_OBJ8_Type"
  Data Type Conversion41/1 -> Bus Creator/41  "FRR_OBJ8_Width"
  Data Type Conversion42/1 -> Bus Creator/42  "FRR_RollingCounter_0x1A6"
  Bus Creator/1 -> SRR_ADCU_FRR_OBJPos4_0x1A6FromOutData/1  "SRR_ADCU_FRR_OBJPos4_0x1A6FromOutData"
  SRR_ADCU_FRR_OBJPos4_0x1A6FromInData/1 -> CAN FD Unpack/1  "SRR_ADCU_FRR_OBJPos4_0x1A6FromInData"
